simulink model "feed_forward2"  (R2023b)
settings: Solver=VariableStepAuto  StartTime=0.0  StopTime=100.0  RelTol=1e-3
settings Model: Creator=86189  LastModifiedBy=86189

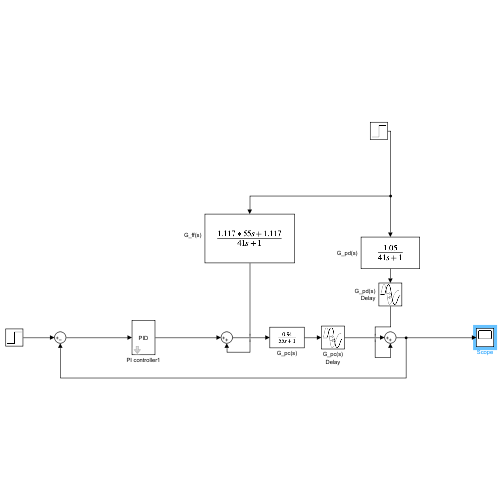
[thumbnail: Simulink's stored preview of the top-level diagram]
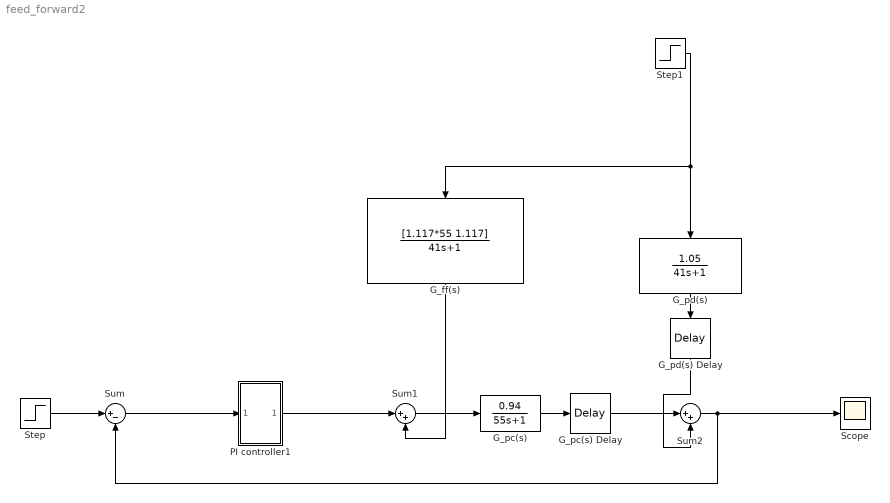
== system feed_forward2 ==
  "G_ff(s) " : TransferFcn  Numerator=[1.117*55 1.117]  Denominator=[41 1]
  G_pc(s) : TransferFcn  Numerator=[0.94]  Denominator=[55 1]
  G_pc(s) Delay : TransportDelay  DelayTime=8
  G_pd(s) : TransferFcn  Numerator=[1.05]  Denominator=[41 1]
  G_pd(s) Delay : TransportDelay  DelayTime=6
  PI controller1 : Subsystem  mask{K_c=5.625, T_u=25}
      mask DialogControl ParameterGroupVar Prompt: 参数
      mask Display: disp('PID')
  Scope : Scope
  Step : Step  SampleTime=0
  Step1 : Step  SampleTime=0
  Sum : Sum  Inputs=|+-
  Sum1 : Sum  Inputs=|++
  Sum2 : Sum  Inputs=|++
  wires:
  G_pc(s)/1 -> G_pc(s) Delay/1
  G_pc(s) Delay/1 -> Sum2/1
  Sum2/1 -> Scope/1, Sum/2
  G_pd(s)/1 -> G_pd(s) Delay/1
  G_pd(s) Delay/1 -> Sum2/2
  Sum1/1 -> G_pc(s)/1
  Step1/1 -> "G_ff(s) "/1, G_pd(s)/1
  Step/1 -> Sum/1
  Sum/1 -> PI controller1/1(In1)
  PI controller1/1(Out1) -> Sum1/1
  "G_ff(s) "/1 -> Sum1/2

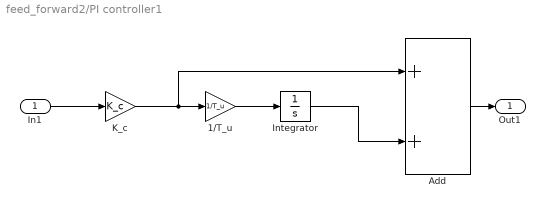
== system feed_forward2/PI controller1 ==
  In1 : Inport
  1/T_u : Gain  Gain=1/T_u
  Add : Sum
  Integrator : Integrator
  K_c : Gain  Gain=K_c
  Out1 : Outport
  wires:
  K_c/1 -> Add/1, 1/T_u/1
  1/T_u/1 -> Integrator/1
  Add/1 -> Out1/1
  In1/1 -> K_c/1
  Integrator/1 -> Add/2
